simulink model "DDSRF"  (Simulink 7.7)
settings: Solver=ode45  StartTime=0.0  StopTime=0.8  RelTol=1e-3
values from neighbouring files (symbols this model uses):
  ki = (wn^2)/Em    [PLL_Init_3approaches.m]    (also in PLL_Init_complete_without_recent_errata.m; approach_comp.m = (wn.^2)./Em; cardan_self_consistent.m; cardan_self_consistent_inbuiltsolve.m)
  kp = 2*del*wn/Em    [PLL_Init_3approaches.m]    (also in PLL_Init_complete_without_recent_errata.m; approach_comp.m = 2.*del.*wn/Em; cardan_self_consistent.m; cardan_self_consistent_inbuiltsolve.m)
  wf = 2*pi*50/sqrt(2)    [PLL_Init_3approaches.m]    (also in PLL_Init_complete_without_recent_errata.m)
libraries: aerolibobsolete x3
settings Model: Creator=Sambhav  LastModifiedBy=Sambhav

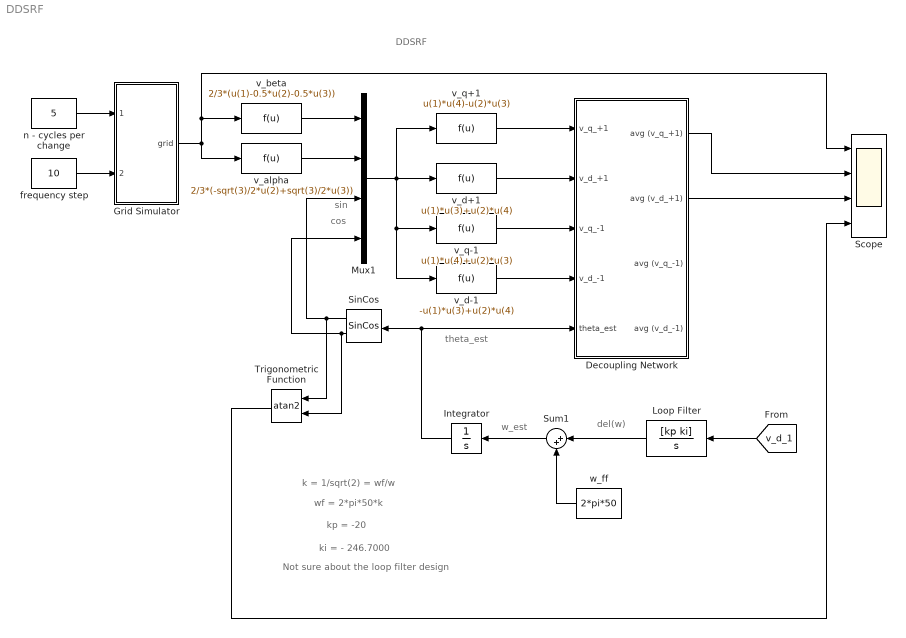
== system DDSRF ==
  note: cos
  note: sin
  note: del(w)
  note: w_est
  note: theta_est
  note: k = 1/sqrt(2) = wf/w
  note: wf = 2*pi*50*k
  note: DDSRF
  note: kp = -20
  note: ki = - 246.7000
  note: Not sure about the loop filter design
  Decoupling Network : Subsystem
  Grid Simulator : Subsystem
  Integrator : Integrator
  Loop Filter : TransferFcn  Numerator=[kp ki]  Denominator=[1 0]
  Mux1 : Mux
  Scope : Scope  NumInputPorts=4
      settings: YMin=-5~-5~-5~-5  YMax=5~5~5~5  SampleInput=on  SampleTime=0.0001
  SinCos : aerolibobsolete/SinCos  SystemSampleTime=-1
  Sum1 : Sum  Inputs=|++
  Trigonometric Function : Trigonometry  Operator=atan2
  frequency step : Constant  Value=10
  n - cycles per change : Constant  Value=5
  v_alpha : Fcn  Expr=2/3*(-sqrt(3)/2*u(2)+sqrt(3)/2*u(3))
  v_beta : Fcn  Expr=2/3*(u(1)-0.5*u(2)-0.5*u(3))
  v_d+1 : Fcn  Expr=u(1)*u(3)+u(2)*u(4)
  v_d-1 : Fcn  Expr=-u(1)*u(3)+u(2)*u(4)
  v_q+1 : Fcn  Expr=u(1)*u(4)-u(2)*u(3)
  v_q-1 : Fcn  Expr=u(1)*u(4)+u(2)*u(3)
  w_ff : Constant  Value=2*pi*50
  wires:
  SinCos/2 -> Mux1/4, Trigonometric Function/2
  SinCos/1 -> Mux1/3, Trigonometric Function/1
  v_alpha/1 -> Mux1/2
  v_beta/1 -> Mux1/1
  v_q+1/1 -> Decoupling Network/1(v_q_+1)
  v_d+1/1 -> Decoupling Network/2(v_d_+1)
  v_q-1/1 -> Decoupling Network/3(v_q_-1)
  v_d-1/1 -> Decoupling Network/4(v_d_-1)
  Mux1/1 -> v_d+1/1, v_q+1/1, v_q-1/1, v_d-1/1
  Loop Filter/1 -> Sum1/1
  Sum1/1 -> Integrator/1
  w_ff/1 -> Sum1/2
  Decoupling Network/2(avg (v_d_+1)) -> Scope/3
  Integrator/1 -> SinCos/1, Decoupling Network/5(theta_est)
  Decoupling Network/1(avg (v_q_+1)) -> Scope/2
  Trigonometric Function/1 -> Scope/4
  n - cycles per change/1 -> Grid Simulator/1(n cycles)
  frequency step/1 -> Grid Simulator/2(freq_step)
  Grid Simulator/1(grid) -> v_alpha/1, v_beta/1, Scope/1
  [v_d_1] -> Loop Filter/1

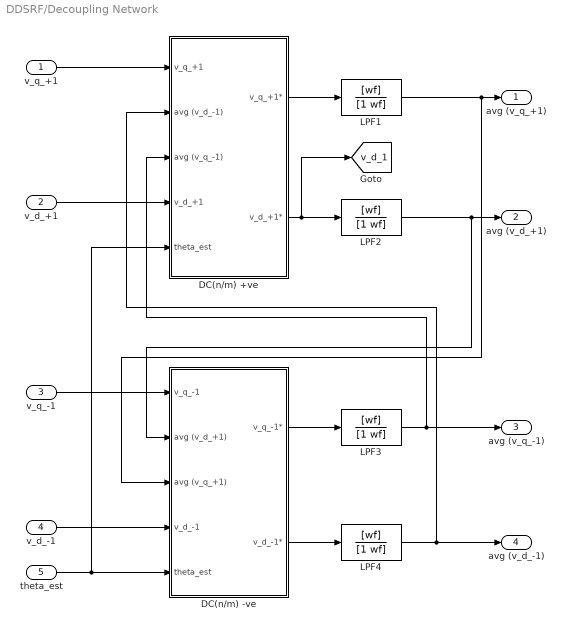
== system DDSRF/Decoupling Network ==
  v_q_+1 : Inport
  v_d_+1 : Inport  Port=2
  v_q_-1 : Inport  Port=3
  v_d_-1 : Inport  Port=4
  theta_est : Inport  Port=5
  DC(n/m) +ve : Subsystem
  DC(n/m) -ve : Subsystem
  LPF{1..4} (4 alike) : TransferFcn  Numerator=[wf]  Denominator=[1 wf]
  avg (v_q_+1) : Outport
  avg (v_d_+1) : Outport  Port=2
  avg (v_q_-1) : Outport  Port=3
  avg (v_d_-1) : Outport  Port=4
  tag scope: v_d_1=global
  wires:
  DC(n/m) +ve/1(v_q_+1*) -> LPF1/1
  DC(n/m) +ve/2(v_d_+1*) -> LPF2/1, [v_d_1]
  DC(n/m) -ve/1(v_q_-1*) -> LPF3/1
  DC(n/m) -ve/2(v_d_-1*) -> LPF4/1
  LPF4/1 -> DC(n/m) +ve/2(avg (v_d_-1)), avg (v_d_-1)/1
  LPF3/1 -> DC(n/m) +ve/3(avg (v_q_-1)), avg (v_q_-1)/1
  LPF2/1 -> DC(n/m) -ve/2(avg (v_d_+1)), avg (v_d_+1)/1
  LPF1/1 -> DC(n/m) -ve/3(avg (v_q_+1)), avg (v_q_+1)/1
  theta_est/1 -> DC(n/m) +ve/5(theta_est), DC(n/m) -ve/5(theta_est)
  v_q_+1/1 -> DC(n/m) +ve/1(v_q_+1)
  v_d_+1/1 -> DC(n/m) +ve/4(v_d_+1)
  v_q_-1/1 -> DC(n/m) -ve/1(v_q_-1)
  v_d_-1/1 -> DC(n/m) -ve/4(v_d_-1)

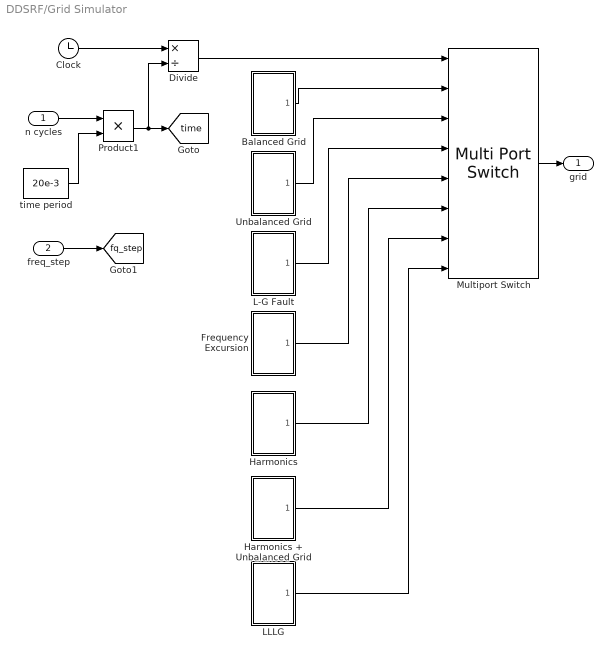
== system DDSRF/Grid Simulator ==
  n cycles : Inport
  freq_step : Inport  Port=2
  Balanced Grid : Subsystem
  Clock : Clock
  Divide : Product  Inputs=*/
  Frequency Excursion : Subsystem
  Harmonics : Subsystem
  Harmonics + Unbalanced Grid : Subsystem
  L-G Fault : Subsystem
  LLLG : Subsystem
  Multiport Switch : MultiPortSwitch  Inputs=7  DiagnosticForDefault=None  zeroidx=off
  Product1 : Product  RndMeth=Zero
  Unbalanced Grid : Subsystem
  time period : Constant  Value=20e-3
  grid : Outport
  tag scope: fq_step=global, time=global
  wires:
  Balanced Grid/1(v_grid) -> Multiport Switch/2
  L-G Fault/1(v_grid) -> Multiport Switch/4
  Frequency Excursion/1(v_grid) -> Multiport Switch/5
  Harmonics/1(v_grid) -> Multiport Switch/6
  Clock/1 -> Divide/1
  time period/1 -> Product1/2
  Product1/1 -> Divide/2, [time]
  Divide/1 -> Multiport Switch/1
  Harmonics + Unbalanced Grid/1(v_grid) -> Multiport Switch/7
  n cycles/1 -> Product1/1
  Multiport Switch/1 -> grid/1
  freq_step/1 -> [fq_step]
  LLLG/1(v_grid) -> Multiport Switch/8
  Unbalanced Grid/1(v_grid) -> Multiport Switch/3

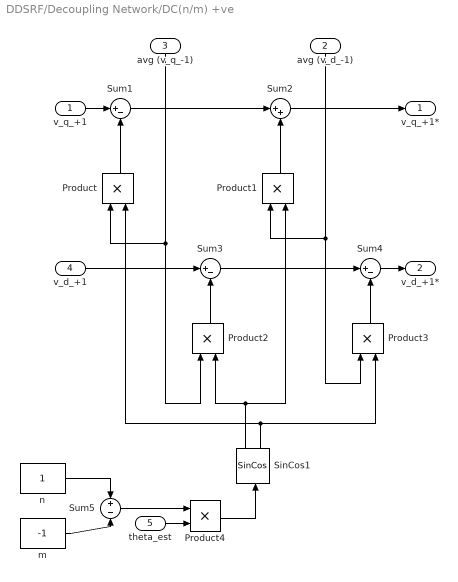
== system DDSRF/Decoupling Network/DC(n/m) +ve ==
  v_q_+1 : Inport
  avg (v_d_-1) : Inport  Port=2
  avg (v_q_-1) : Inport  Port=3
  v_d_+1 : Inport  Port=4
  theta_est : Inport  Port=5
  Product{,1..4} (5 alike) : Product  RndMeth=Zero
  SinCos1 : aerolibobsolete/SinCos  SystemSampleTime=-1
  Sum1 : Sum  Inputs=|+-
  Sum2 : Sum  Inputs=|++
  Sum3 : Sum  Inputs=|+-
  Sum4 : Sum  Inputs=|+-
  Sum5 : Sum  Inputs=+|-
  m : Constant  Value=-1
  n : Constant
  v_q_+1* : Outport
  v_d_+1* : Outport  Port=2
  wires:
  Product/1 -> Sum1/2
  SinCos1/2 -> Product/2, Product3/2
  Sum1/1 -> Sum2/1
  Product1/1 -> Sum2/2
  SinCos1/1 -> Product1/2, Product2/2
  Product2/1 -> Sum3/2
  Sum3/1 -> Sum4/1
  Product3/1 -> Sum4/2
  avg (v_q_-1)/1 -> Product/1, Product2/1
  avg (v_d_-1)/1 -> Product1/1, Product3/1
  n/1 -> Sum5/1
  Sum5/1 -> Product4/1
  Product4/1 -> SinCos1/1
  m/1 -> Sum5/2
  v_q_+1/1 -> Sum1/1
  Sum2/1 -> v_q_+1*/1
  v_d_+1/1 -> Sum3/1
  Sum4/1 -> v_d_+1*/1
  theta_est/1 -> Product4/2

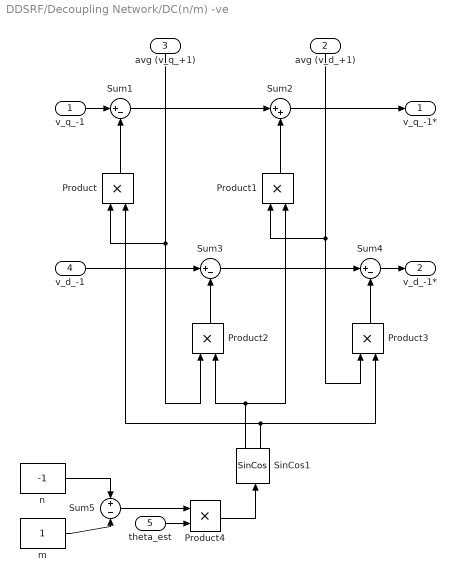
== system DDSRF/Decoupling Network/DC(n/m) -ve ==
  v_q_-1 : Inport
  avg (v_d_+1) : Inport  Port=2
  avg (v_q_+1) : Inport  Port=3
  v_d_-1 : Inport  Port=4
  theta_est : Inport  Port=5
  Product{,1..4} (5 alike) : Product  RndMeth=Zero
  SinCos1 : aerolibobsolete/SinCos  SystemSampleTime=-1
  Sum1 : Sum  Inputs=|+-
  Sum2 : Sum  Inputs=|++
  Sum3 : Sum  Inputs=|+-
  Sum4 : Sum  Inputs=|+-
  Sum5 : Sum  Inputs=+|-
  m : Constant
  n : Constant  Value=-1
  v_q_-1* : Outport
  v_d_-1* : Outport  Port=2
  wires:
  theta_est/1 -> Product4/2
  Sum4/1 -> v_d_-1*/1
  v_d_-1/1 -> Sum3/1
  Sum2/1 -> v_q_-1*/1
  v_q_-1/1 -> Sum1/1
  m/1 -> Sum5/2
  Product4/1 -> SinCos1/1
  Sum5/1 -> Product4/1
  n/1 -> Sum5/1
  avg (v_d_+1)/1 -> Product3/1, Product1/1
  avg (v_q_+1)/1 -> Product2/1, Product/1
  Product3/1 -> Sum4/2
  Sum3/1 -> Sum4/1
  Product2/1 -> Sum3/2
  SinCos1/1 -> Product2/2, Product1/2
  Product1/1 -> Sum2/2
  Sum1/1 -> Sum2/1
  SinCos1/2 -> Product3/2, Product/2
  Product/1 -> Sum1/2

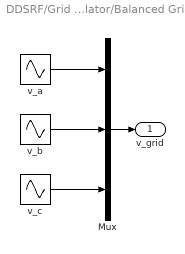
== system DDSRF/Grid Simulator/Balanced Grid ==
  Mux : Mux  Inputs=3
  v_a : Sin  Amplitude=230*sqrt(2)  Frequency=2*pi*50  Phase=pi/2  SampleTime=0
  v_b : Sin  Amplitude=230*sqrt(2)  Frequency=2*pi*50  Phase=pi/2-2*pi/3  SampleTime=0
  v_c : Sin  Amplitude=230*sqrt(2)  Frequency=2*pi*50  Phase=pi/2+2*pi/3  SampleTime=0
  v_grid : Outport
  wires:
  v_a/1 -> Mux/1
  v_b/1 -> Mux/2
  v_c/1 -> Mux/3
  Mux/1 -> v_grid/1

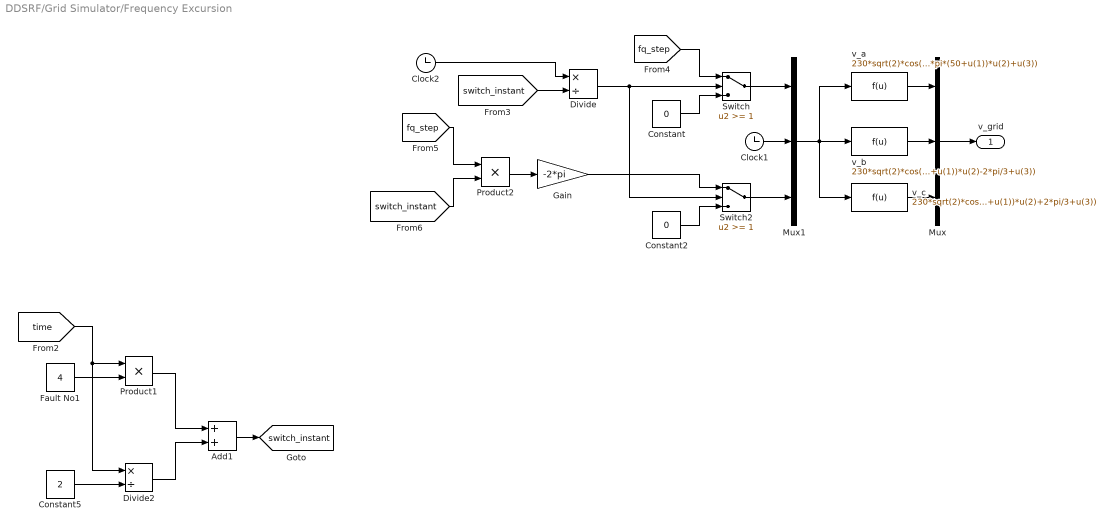
== system DDSRF/Grid Simulator/Frequency Excursion ==
  Add1 : Sum
  Clock1 : Clock
      settings: Decimation=10
  Clock2 : Clock
      settings: Decimation=10
  Constant : Constant  Value=0
  Constant2 : Constant  Value=0
  Constant5 : Constant  Value=2
  Divide : Product  Inputs=*/
  Divide2 : Product  Inputs=*/
  Fault No1 : Constant  Value=4
  Gain : Gain  Gain=-2*pi
  Mux : Mux  Inputs=3
  Mux1 : Mux  Inputs=3
  Product1 : Product  RndMeth=Zero
  Product2 : Product  RndMeth=Zero
  Switch : Switch  Threshold=1
  Switch2 : Switch  Threshold=1
  v_a : Fcn  Expr=230*sqrt(2)*cos(2*pi*(50+u(1))*u(2)+u(3))
  v_b : Fcn  Expr=230*sqrt(2)*cos(2*pi*(50+u(1))*u(2)-2*pi/3+u(3))
  v_c : Fcn  Expr=230*sqrt(2)*cos(2*pi*(50+u(1))*u(2)+2*pi/3+u(3))
  v_grid : Outport
  tag scope: switch_instant=global
  wires:
  [fq_step] -> Switch/1
  Constant/1 -> Switch/3
  Mux1/1 -> v_a/1, v_b/1, v_c/1
  v_a/1 -> Mux/1
  v_b/1 -> Mux/2
  v_c/1 -> Mux/3
  Constant2/1 -> Switch2/3
  Switch2/1 -> Mux1/3
  Gain/1 -> Switch2/1
  [time] -> Divide2/1, Product1/1
  Fault No1/1 -> Product1/2
  Product1/1 -> Add1/1
  Constant5/1 -> Divide2/2
  Divide2/1 -> Add1/2
  Mux/1 -> v_grid/1
  Switch/1 -> Mux1/1
  Clock2/1 -> Divide/1
  Add1/1 -> [switch_instant]
  [switch_instant] -> Divide/2
  Divide/1 -> Switch/2, Switch2/2
  [fq_step] -> Product2/1
  [switch_instant] -> Product2/2
  Product2/1 -> Gain/1
  Clock1/1 -> Mux1/2

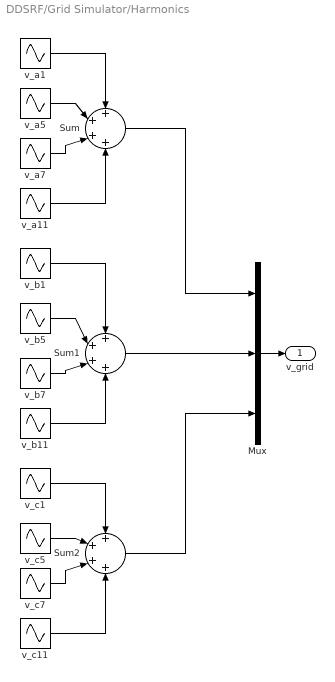
== system DDSRF/Grid Simulator/Harmonics ==
  Mux : Mux  Inputs=3
  Sum : Sum  Inputs=+|+|+|+
  Sum1 : Sum  Inputs=+|+|+|+
  Sum2 : Sum  Inputs=+|+|+|+
  v_a1 : Sin  Amplitude=230*sqrt(2)  Frequency=2*pi*50  Phase=pi/2  SampleTime=0
  v_a11 : Sin  Amplitude=230*sqrt(2)/11  Frequency=2*pi*50*11  Phase=pi/2  SampleTime=0
  v_a5 : Sin  Amplitude=230*sqrt(2)/5  Frequency=2*pi*50*5  Phase=pi/2  SampleTime=0
  v_a7 : Sin  Amplitude=230*sqrt(2)/7  Frequency=2*pi*50*7  Phase=pi/2  SampleTime=0
  v_b1 : Sin  Amplitude=230*sqrt(2)  Frequency=2*pi*50  Phase=pi/2-2*pi/3  SampleTime=0
  v_b11 : Sin  Amplitude=230*sqrt(2)/11  Frequency=2*pi*50*11  Phase=pi/2-2*pi/3  SampleTime=0
  v_b5 : Sin  Amplitude=230*sqrt(2)/5  Frequency=2*pi*50*5  Phase=pi/2-2*pi/3  SampleTime=0
  v_b7 : Sin  Amplitude=230*sqrt(2)/7  Frequency=2*pi*50*7  Phase=pi/2-2*pi/3  SampleTime=0
  v_c1 : Sin  Amplitude=230*sqrt(2)  Frequency=2*pi*50  Phase=pi/2+2*pi/3  SampleTime=0
  v_c11 : Sin  Amplitude=230*sqrt(2)/11  Frequency=2*pi*50*11  Phase=pi/2+2*pi/3  SampleTime=0
  v_c5 : Sin  Amplitude=230*sqrt(2)/5  Frequency=2*pi*50*5  Phase=pi/2+2*pi/3  SampleTime=0
  v_c7 : Sin  Amplitude=230*sqrt(2)/7  Frequency=2*pi*50*7  Phase=pi/2+2*pi/3  SampleTime=0
  v_grid : Outport
  wires:
  Mux/1 -> v_grid/1
  v_a1/1 -> Sum/1
  v_a5/1 -> Sum/2
  v_a7/1 -> Sum/3
  v_a11/1 -> Sum/4
  v_b1/1 -> Sum1/1
  v_b11/1 -> Sum1/4
  v_b5/1 -> Sum1/2
  v_b7/1 -> Sum1/3
  v_c1/1 -> Sum2/1
  v_c5/1 -> Sum2/2
  v_c7/1 -> Sum2/3
  v_c11/1 -> Sum2/4
  Sum/1 -> Mux/1
  Sum1/1 -> Mux/2
  Sum2/1 -> Mux/3

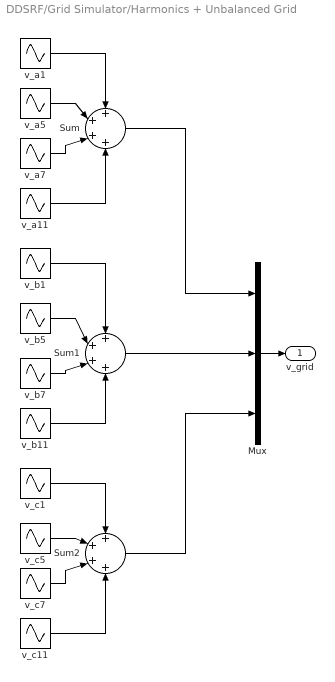
== system DDSRF/Grid Simulator/Harmonics + Unbalanced Grid ==
  Mux : Mux  Inputs=3
  Sum : Sum  Inputs=+|+|+|+
  Sum1 : Sum  Inputs=+|+|+|+
  Sum2 : Sum  Inputs=+|+|+|+
  v_a1 : Sin  Amplitude=230*sqrt(2)  Frequency=2*pi*50  Phase=pi/2  SampleTime=0
  v_a11 : Sin  Amplitude=230*sqrt(2)/11  Frequency=2*pi*50*11  Phase=pi/2  SampleTime=0
  v_a5 : Sin  Amplitude=230*sqrt(2)/5  Frequency=2*pi*50*5  Phase=pi/2  SampleTime=0
  v_a7 : Sin  Amplitude=230*sqrt(2)/7  Frequency=2*pi*50*7  Phase=pi/2  SampleTime=0
  v_b1 : Sin  Amplitude=200*sqrt(2)  Frequency=2*pi*50  Phase=pi/2-2*pi/3+pi/6  SampleTime=0
  v_b11 : Sin  Amplitude=220*sqrt(2)/11  Frequency=2*pi*50*11  Phase=pi/2-2*pi/3+pi/6  SampleTime=0
  v_b5 : Sin  Amplitude=200*sqrt(2)/5  Frequency=2*pi*50*5  Phase=pi/2-2*pi/3+pi/6  SampleTime=0
  v_b7 : Sin  Amplitude=200*sqrt(2)/7  Frequency=2*pi*50*7  Phase=pi/2-2*pi/3+pi/6  SampleTime=0
  v_c1 : Sin  Amplitude=210*sqrt(2)  Frequency=2*pi*50  Phase=pi/2+2*pi/3-pi/18  SampleTime=0
  v_c11 : Sin  Amplitude=210*sqrt(2)/11  Frequency=2*pi*50*11  Phase=pi/2+2*pi/3-pi/18  SampleTime=0
  v_c5 : Sin  Amplitude=210*sqrt(2)/5  Frequency=2*pi*50*5  Phase=pi/2+2*pi/3-pi/18  SampleTime=0
  v_c7 : Sin  Amplitude=210*sqrt(2)/7  Frequency=2*pi*50*7  Phase=pi/2+2*pi/3-pi/18  SampleTime=0
  v_grid : Outport
  wires:
  Sum2/1 -> Mux/3
  Sum1/1 -> Mux/2
  Sum/1 -> Mux/1
  v_c11/1 -> Sum2/4
  v_c7/1 -> Sum2/3
  v_c5/1 -> Sum2/2
  v_c1/1 -> Sum2/1
  v_b7/1 -> Sum1/3
  v_b5/1 -> Sum1/2
  v_b11/1 -> Sum1/4
  v_b1/1 -> Sum1/1
  v_a11/1 -> Sum/4
  v_a7/1 -> Sum/3
  v_a5/1 -> Sum/2
  v_a1/1 -> Sum/1
  Mux/1 -> v_grid/1

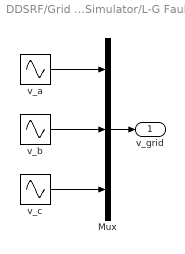
== system DDSRF/Grid Simulator/L-G Fault ==
  Mux : Mux  Inputs=3
  v_a : Sin  Amplitude=230*sqrt(2)  Frequency=2*pi*50  Phase=pi/2  SampleTime=0
  v_b : Sin  Amplitude=10  Frequency=2*pi*50  Phase=pi/2-2*pi/3  SampleTime=0
  v_c : Sin  Amplitude=230*sqrt(2)  Frequency=2*pi*50  Phase=pi/2+2*pi/3  SampleTime=0
  v_grid : Outport
  wires:
  Mux/1 -> v_grid/1
  v_c/1 -> Mux/3
  v_b/1 -> Mux/2
  v_a/1 -> Mux/1

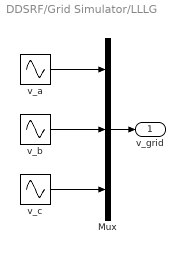
== system DDSRF/Grid Simulator/LLLG ==
  Mux : Mux  Inputs=3
  v_a : Sin  Amplitude=0  Frequency=0  SampleTime=0
  v_b : Sin  Amplitude=0  Frequency=0  SampleTime=0
  v_c : Sin  Amplitude=0  Frequency=0  SampleTime=0
  v_grid : Outport
  wires:
  Mux/1 -> v_grid/1
  v_c/1 -> Mux/3
  v_b/1 -> Mux/2
  v_a/1 -> Mux/1

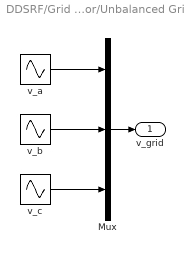
== system DDSRF/Grid Simulator/Unbalanced Grid ==
  Mux : Mux  Inputs=3
  v_a : Sin  Amplitude=230*sqrt(2)  Frequency=2*pi*50  Phase=pi/2  SampleTime=0
  v_b : Sin  Amplitude=200*sqrt(2)  Frequency=2*pi*50  Phase=pi/2-2*pi/3+pi/6  SampleTime=0
  v_c : Sin  Amplitude=210*sqrt(2)  Frequency=2*pi*50  Phase=pi/2+2*pi/3-pi/18  SampleTime=0
  v_grid : Outport
  wires:
  v_a/1 -> Mux/1
  v_b/1 -> Mux/2
  v_c/1 -> Mux/3
  Mux/1 -> v_grid/1
